simulink model "E5S_Prueba_Simulacion"  (R2020a)
settings: Solver=VariableStepAuto  StartTime=0.0  StopTime=0.5  RelTol=1e-3
undefined symbols (not defined in the file): J_a, K, K_ml_arb, K_ml_bos, K_ml_pol, K_ml_svr
libraries: fl_lib x20, nesl_utility x20, ee_lib x15
settings Model: Creator=Luis Angel  LastModifiedBy=Luis Angel

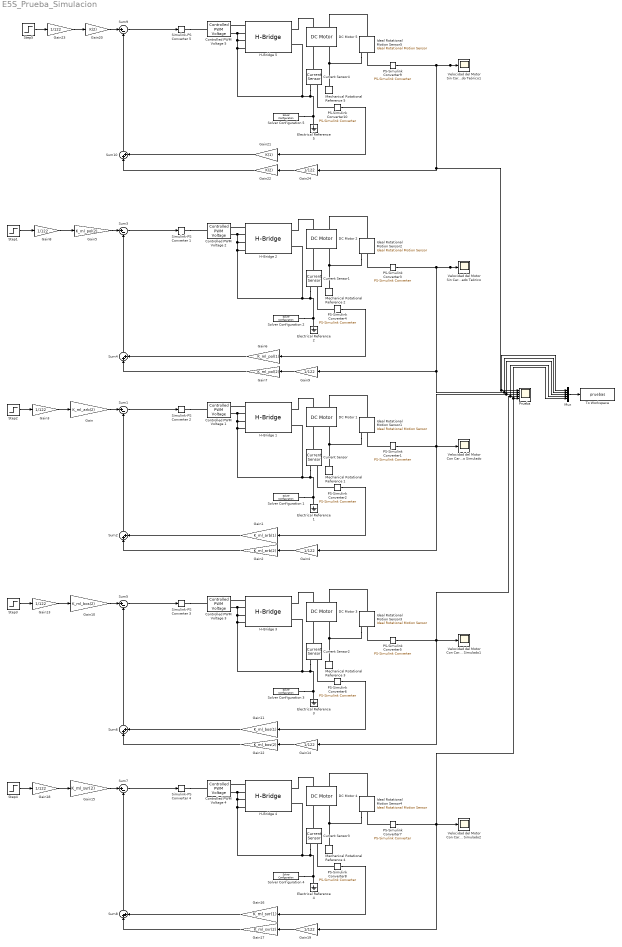
== system E5S_Prueba_Simulacion ==
   Ideal Rotational Motion Sensor{1..5} (5 alike) : fl_lib/Mechanical/Mechanical Sensors/Ideal Rotational Motion Sensor  wrap_angle=simscape.enum.onoff.off  offset=0 rad
   PS-Simulink Converter{1,3,5,7,9} (5 alike) : nesl_utility/PS-Simulink Converter  PhysicalDomain=network_engine_domain  SubClassName=ps_output  LeftPortType=input  RightPortType=output  PseudoPeriodic=off  Frequencies=[]  Unit=rad/s  AffineConversion=on
   PS-Simulink Converter{2,4,6,8,10} (5 alike) : nesl_utility/PS-Simulink Converter  PhysicalDomain=network_engine_domain  SubClassName=ps_output  LeftPortType=input  RightPortType=output  PseudoPeriodic=off  Frequencies=[]  Unit=A  AffineConversion=on
  Controlled PWM Voltage {1..5} (5 alike) : ee_lib/Integrated Circuits/Controlled PWM Voltage  F=1000 Hz  TD=0 s  pulse_width_offset=0 s  pulse_min=0 s  Vmin=0 V  Vmax=5 V  Vm=5 V  pwm_or_av=2  event_type=1  sample_time=1e-6 s  u_min=0  u_max=1
      settings: InternalSimscapePortConfiguration="{\"Bottom\":[],\"Left\":[{\"id\":\"u\",\"label\":\"u\",\"type\":\"input\"}],\"Right\":[{\"id\":\"p2\",\"label\":\"PWM\",\"type\":\"foundation.electrical.electrical\"},{\"id\":\"n2\",\"label\":\"REF\",\"type\":\"foundation.electrical.electrical\"}],\"Top\":[]}"
  Current Sensor{,1..4} (5 alike) : fl_lib/Electrical/Electrical Sensors/Current Sensor
  DC Motor {1..5} (5 alike) : ee_lib/Electromechanical/Brushed Motors/DC Motor  field_option=ee.enum.field_option.pm  Rf=100 Ohm  Lf=1 H  Laf=0.15 H  If0=0 A  parameterization=ee.enum.dcparam_option.circuit_param  Ra=R Ohm  La=L H  emf_or_torque=ee.enum.emf_or_torque.kv  Kv=km V/(rad/s)  Ki=6.876e-4 N*m/A  T_stall=0.24e-3 N*m  w_max=19100 rpm  w_rated=15000 rpm  P_rated=0.08 W  V_rated=1.5 V  J=J_a kg*m^2  lam_param=ee.enum.lam_param.damping  lam=B N*m/(rad/s)  i_noload=0 A  V_i_noload=1.5 V  speed0=0 rad/s  alpha=3.93e-3 1/K  Tmeas=25 degC  thermal_mass=100 J/K  initial_temperature=25 degC
  Electrical Reference {1..5} (5 alike) : fl_lib/Electrical/Electrical Elements/Electrical Reference
      settings: SourceProductBaseCode=MT,SS
  Gain : Gain  Gain=K_ml_arb(2)
  Gain1 : Gain  Gain=K_ml_arb(1)
  Gain10 : Gain  Gain=K_ml_bos(2)
  Gain11 : Gain  Gain=K_ml_bos(1)
  Gain12 : Gain  Gain=K_ml_bos(2)
  Gain{3..4,8..9,13..14,18..19,23..24} (10 alike) : Gain  Gain=1/122
  Gain15 : Gain  Gain=K_ml_svr(2)
  Gain16 : Gain  Gain=K_ml_svr(1)
  Gain17 : Gain  Gain=K_ml_svr(2)
  Gain2 : Gain  Gain=K_ml_arb(2)
  Gain20 : Gain  Gain=K(2)
  Gain21 : Gain  Gain=K(1)
  Gain22 : Gain  Gain=K(2)
  Gain5 : Gain  Gain=K_ml_pol(2)
  Gain6 : Gain  Gain=K_ml_pol(1)
  Gain7 : Gain  Gain=K_ml_pol(2)
  H-Bridge {1..5} (5 alike) : ee_lib/Semiconductors & Converters/Converters/H-Bridge  supply_ports=ee.enum.supply_ports.hidesupply  Venable=2.5 V  Vmax=5 V  Vreverse=2.5 V  Vbrake=2.5 V  Vm=Va V  pwm_or_av=ee.enum.pwm_or_av.averaged  regenerative_braking_mode=ee.enum.converters.regenerative_braking_mode.always_enabled  discontinuous=ee.enum.current_profile.continuous  freewheeling_mode=ee.enum.converters.freewheeling_mode.one_switch_one_diode  Ron=0.1 Ohm  Don=0.05 Ohm  Goff=1e-6 S  Rload=10 Ohm  Lload=1e-5 H  F=10 kHz  thermal_mass=100 J/K  initial_temperature=298.15 K  Ron2=0.1 Ohm  Don2=0.05 Ohm  Tmeas=298.15 K  Tmeas2=398.15 K
  Mechanical Rotational Reference {1..5} (5 alike) : fl_lib/Mechanical/Rotational Elements/Mechanical Rotational Reference
  Mux : Mux  Inputs=5
  Prueba : Scope  NumInputPorts=5
  Simulink-PS Converter {1..5} (5 alike) : nesl_utility/Simulink-PS Converter  PhysicalDomain=network_engine_domain  SubClassName=ps_input  LeftPortType=input  RightPortType=output  PseudoPeriodic=off  Frequencies=[]  NoiseDistribution=none  NoiseParameters=[]  Unit=1  AffineConversion=off  FilteringAndDerivatives=provide  SimscapeFilterOrder=1  InputFilterTimeConstant=0.001  UdotUserProvided=0
  Solver Configuration {1..5} (5 alike) : nesl_utility/Solver Configuration  PhysicalDomain=network_engine_domain  SubClassName=solver  LeftPortType=input  RightPortType=generic  Tones=[]  Harmonics=[]  SimulateNoise=off  Profile=off  UseLocalSampling=off  EnableSwitchedLinearOptims=on  FrequencyDomain=off  UseCCode=off  RelTol=0.001  AbsTol=1e-06  MinStep=1e-09  ToWorkspace=off  RevertToSquareIcSolve=off  NumHomotopyIterations=100  PhasorMode=off  PhasorModeNumHarmonics=1  DoDC=off  ResidualTolerance=1e-09  UseLocalSolver=off  LocalSolverChoice=NE_BACKWARD_EULER_ADVANCER  LocalSolverSampleTime=0.001  DoFixedCost=off  MaxNonlinIter=3  MaxModeIter=2  LinearAlgebra=auto  EquationFormulation=NE_TIME_EF  DelaysMemoryBudget=1024  AutomaticFiltering=on  FilteringTimeConstant=0.001  PartitionStorageMethod=AS_NEEDED  PartitionMemoryBudget=1024  PartitionMethod=ROBUST
  Step{1..5} (5 alike) : Step  Time=0  After=52.46  SampleTime=0
  Sum{1,3,5,7,9} (5 alike) : Sum  Inputs=|+-
  Sum{2,4,6,8,10} (5 alike) : Sum  Inputs=|++
  To Workspace : ToWorkspace  VariableName=pruebas  SaveFormat=Timeseries  SampleTime=0.00001
  Velocidad del Motor Con Carga Controlado Simulado : Scope
  Velocidad del Motor Con Carga Controlado Simulado1 : Scope
  Velocidad del Motor Con Carga Controlado Simulado2 : Scope
  Velocidad del Motor Sin Carga Controlado Teórico : Scope
  Velocidad del Motor Sin Carga Controlado Teórico1 : Scope
  wires:
  Gain4/1 -> Gain2/1
  Gain3/1 -> Gain/1
  Sum2/1 -> Sum1/2
  Gain/1 -> Sum1/1
  Sum1/1 -> Simulink-PS Converter 2/1
  Step2/1 -> Gain3/1
  Gain1/1 -> Sum2/2
  " PS-Simulink Converter2"/1 -> Gain1/1
  Gain2/1 -> Sum2/1
  " PS-Simulink Converter1"/1 -> Mux/3, Prueba/3, Gain4/1, Velocidad del Motor Con Carga Controlado Simulado/1
  " PS-Simulink Converter3"/1 -> Mux/2, Prueba/2, Gain9/1, Velocidad del Motor Sin Carga Controlado Teórico/1
  Gain9/1 -> Gain7/1
  Sum3/1 -> Simulink-PS Converter 1/1
  Gain6/1 -> Sum4/2
  Gain5/1 -> Sum3/1
  Step1/1 -> Gain8/1
  " PS-Simulink Converter4"/1 -> Gain6/1
  Sum4/1 -> Sum3/2
  Gain8/1 -> Gain5/1
  Gain7/1 -> Sum4/1
  Sum6/1 -> Sum5/2
  " PS-Simulink Converter6"/1 -> Gain11/1
  Sum5/1 -> Simulink-PS Converter 3/1
  Gain11/1 -> Sum6/2
  Gain13/1 -> Gain10/1
  " PS-Simulink Converter5"/1 -> Prueba/4, Mux/4, Gain14/1, Velocidad del Motor Con Carga Controlado Simulado1/1
  Gain14/1 -> Gain12/1
  Gain10/1 -> Sum5/1
  Gain12/1 -> Sum6/1
  Step3/1 -> Gain13/1
  Gain18/1 -> Gain15/1
  Gain19/1 -> Gain17/1
  Step4/1 -> Gain18/1
  Gain17/1 -> Sum8/1
  Gain15/1 -> Sum7/1
  " PS-Simulink Converter7"/1 -> Prueba/5, Mux/5, Velocidad del Motor Con Carga Controlado Simulado2/1, Gain19/1
  Gain16/1 -> Sum8/2
  Sum7/1 -> Simulink-PS Converter 4/1
  " PS-Simulink Converter8"/1 -> Gain16/1
  Sum8/1 -> Sum7/2
  " PS-Simulink Converter10"/1 -> Gain21/1
  Gain22/1 -> Sum10/1
  Gain20/1 -> Sum9/1
  Sum10/1 -> Sum9/2
  Gain24/1 -> Gain22/1
  Gain21/1 -> Sum10/2
  Sum9/1 -> Simulink-PS Converter 5/1
  Gain23/1 -> Gain20/1
  Step5/1 -> Gain23/1
  " PS-Simulink Converter9"/1 -> Mux/1, Prueba/1, Gain24/1, Velocidad del Motor Sin Carga Controlado Teórico1/1
  Mux/1 -> To Workspace/1
  connections:
  Mechanical Rotational Reference 1/LConn1 -- " Ideal Rotational Motion Sensor1"/RConn1 -- DC Motor 1/RConn2
  Controlled PWM Voltage 1/RConn2 -- H-Bridge 1/RConn2 -- Solver Configuration 1/RConn1 -- Electrical Reference 1/LConn1 -- Current Sensor/RConn2 -- H-Bridge 1/LConn4 -- H-Bridge 1/LConn3 -- H-Bridge 1/LConn2
  Current Sensor/LConn1 -- DC Motor 1/RConn1
  H-Bridge 1/LConn1 -- Controlled PWM Voltage 1/RConn1
  " PS-Simulink Converter1"/LConn1 -- " Ideal Rotational Motion Sensor1"/RConn2
  Simulink-PS Converter 2/RConn1 -- Controlled PWM Voltage 1/LConn1
  " Ideal Rotational Motion Sensor1"/LConn1 -- DC Motor 1/LConn2
  " PS-Simulink Converter2"/LConn1 -- Current Sensor/RConn1
  DC Motor 1/LConn1 -- H-Bridge 1/RConn1
  H-Bridge 2/LConn3 -- Controlled PWM Voltage 2/RConn2 -- H-Bridge 2/LConn2 -- H-Bridge 2/RConn2 -- Solver Configuration 2/RConn1 -- Electrical Reference 2/LConn1 -- Current Sensor1/RConn2 -- H-Bridge 2/LConn4
  DC Motor 2/RConn2 -- Mechanical Rotational Reference 2/LConn1 -- " Ideal Rotational Motion Sensor2"/RConn1
  Current Sensor1/LConn1 -- DC Motor 2/RConn1
  Simulink-PS Converter 1/RConn1 -- Controlled PWM Voltage 2/LConn1
  " PS-Simulink Converter3"/LConn1 -- " Ideal Rotational Motion Sensor2"/RConn2
  " PS-Simulink Converter4"/LConn1 -- Current Sensor1/RConn1
  " Ideal Rotational Motion Sensor2"/LConn1 -- DC Motor 2/LConn2
  H-Bridge 2/LConn1 -- Controlled PWM Voltage 2/RConn1
  DC Motor 2/LConn1 -- H-Bridge 2/RConn1
  H-Bridge 3/LConn3 -- Controlled PWM Voltage 3/RConn2 -- H-Bridge 3/LConn2 -- H-Bridge 3/RConn2 -- Solver Configuration 3/RConn1 -- Electrical Reference 3/LConn1 -- Current Sensor2/RConn2 -- H-Bridge 3/LConn4
  DC Motor 3/RConn2 -- Mechanical Rotational Reference 3/LConn1 -- " Ideal Rotational Motion Sensor3"/RConn1
  DC Motor 3/LConn1 -- H-Bridge 3/RConn1
  " PS-Simulink Converter6"/LConn1 -- Current Sensor2/RConn1
  " PS-Simulink Converter5"/LConn1 -- " Ideal Rotational Motion Sensor3"/RConn2
  Simulink-PS Converter 3/RConn1 -- Controlled PWM Voltage 3/LConn1
  " Ideal Rotational Motion Sensor3"/LConn1 -- DC Motor 3/LConn2
  Current Sensor2/LConn1 -- DC Motor 3/RConn1
  H-Bridge 3/LConn1 -- Controlled PWM Voltage 3/RConn1
  H-Bridge 4/LConn3 -- Controlled PWM Voltage 4/RConn2 -- H-Bridge 4/LConn2 -- H-Bridge 4/RConn2 -- Solver Configuration 4/RConn1 -- Electrical Reference 4/LConn1 -- Current Sensor3/RConn2 -- H-Bridge 4/LConn4
  DC Motor 4/RConn2 -- Mechanical Rotational Reference 4/LConn1 -- " Ideal Rotational Motion Sensor4"/RConn1
  DC Motor 4/LConn1 -- H-Bridge 4/RConn1
  " Ideal Rotational Motion Sensor4"/LConn1 -- DC Motor 4/LConn2
  " PS-Simulink Converter8"/LConn1 -- Current Sensor3/RConn1
  H-Bridge 4/LConn1 -- Controlled PWM Voltage 4/RConn1
  Current Sensor3/LConn1 -- DC Motor 4/RConn1
  " PS-Simulink Converter7"/LConn1 -- " Ideal Rotational Motion Sensor4"/RConn2
  Simulink-PS Converter 4/RConn1 -- Controlled PWM Voltage 4/LConn1
  H-Bridge 5/LConn4 -- H-Bridge 5/LConn3 -- Controlled PWM Voltage 5/RConn2 -- H-Bridge 5/LConn2 -- H-Bridge 5/RConn2 -- Solver Configuration 5/RConn1 -- Electrical Reference 5/LConn1 -- Current Sensor4/RConn2
  " Ideal Rotational Motion Sensor5"/RConn1 -- DC Motor 5/RConn2 -- Mechanical Rotational Reference 5/LConn1
  " Ideal Rotational Motion Sensor5"/LConn1 -- DC Motor 5/LConn2
  Simulink-PS Converter 5/RConn1 -- Controlled PWM Voltage 5/LConn1
  H-Bridge 5/LConn1 -- Controlled PWM Voltage 5/RConn1
  " PS-Simulink Converter9"/LConn1 -- " Ideal Rotational Motion Sensor5"/RConn2
  DC Motor 5/LConn1 -- H-Bridge 5/RConn1
  " PS-Simulink Converter10"/LConn1 -- Current Sensor4/RConn1
  Current Sensor4/LConn1 -- DC Motor 5/RConn1
